simulink model "CLAHEExample"  (R2019b)
settings: Solver=FixedStepDiscrete  StartTime=0.0  StopTime=402*324  FixedStep=1  RelTol=1e-3
PreLoadFcn:
  | % Initialize input image size
  | img = [240 320];
  | 
  | % Number of tiles fixed to 8 x 8
  | numTiles = [8 8];
  | 
  | % Initialize clip limit
  | normClipLimit  = 0.01;
  | 
  | % Number of Bins
  | numBins = 256;
  | 
  | dimI = [240 320] ;
  | 
  | dimTiles = dimI ./ numTiles;
  | 
  | numPixInTile = prod(dimTiles);
  | 
  | minClipLimit = ceil(numPixInTile/numBins);
  | 
  | clipLimit = minClipLimit + round(normClipLimit*(numPixInTile-minClipLimit));
  | 
  | % Initialize value for 1-D lookup table
  | tabVal = uint8(floor(numBins./(1:numBins-1)));
  | 
  | % Initialize wordlength and fractionlength
  | normFact1 = fi(1/(dimTiles(1)*dimTiles(2)/4),0);
  | 
  | normFact2 = fi(1/(prod(dimTiles)/2),0);
  | 
  | normFact3 = fi(1/(prod(dimTiles)),0);
  | 
  | grayxval = (numBins-1)/numPixInTile;
  | fi_grayxval = fi(grayxval,0);
InitFcn:
  | img = imread(get_param('CLAHEExample/inputImage','FileName'));
  | %img = [240 320];
  | numTiles = [8 8];
  | 
  | normClipLimit = str2double(get_param('CLAHEExample/CLAHEHDLAlgorithm','normClipLimit'));
  | 
  | numBins = 256;
  | 
  | dimI = size(img);
  | 
  | dimTiles = dimI ./ numTiles;
  | 
  | numPixInTile = prod(dimTiles);
  | 
  | minClipLimit = ceil(numPixInTile/numBins);
  | 
  | clipLimit = minClipLimit + round(normClipLimit*(numPixInTile-minClipLimit));
  | 
  | tabVal = uint8(floor(numBins./(1:numBins-1)));
  | 
  | normFact1 = fi(1/(dimTiles(1)*dimTiles(2)/4),0);
  | 
  | normFact2 = fi(1/(prod(dimTiles)/2),0);
  | 
  | normFact3 = fi(1/(prod(dimTiles)),0);
  | 
  | grayxval = (numBins-1)/numPixInTile;
  | fi_grayxval = fi(grayxval,0);
libraries: simulink x64, hdlsllib x46, visionhdlutilities x9, visionhdlstatistics x2, visionhdlio x2, visionsources x1
(part 2 of 3)

== system CLAHEExample/CLAHEHDLAlgorithm/tileGeneration/Subsystem ==
  In1 : Inport
  In2 : Inport  Port=2
  In3 : Inport  Port=3
  In4 : Inport  Port=4
  In5 : Inport  Port=5
  In6 : Inport  Port=6
  In7 : Inport  Port=7
  In8 : Inport  Port=8
  In9 : Inport  Port=9
  Multiport Switch{1..5} (5 alike) : MultiPortSwitch  Inputs=8
  Pixel Control Bus Creator : visionhdlutilities/Pixel Control Bus Creator
      settings: SourceProductName=Vision HDL Toolbox  SourceProductBaseCode=VT
  Pixel Control Bus Selector{,1..7} (8 alike) : BusSelector  OutputSignals=hStart,hEnd,vStart,vEnd,valid
  Out1 : Outport  VectorParamsAs1DForOutWhenUnconnected=off
  wires:
  In3/1 -> Pixel Control Bus Selector1/1
  In2/1 -> Pixel Control Bus Selector/1
  In4/1 -> Pixel Control Bus Selector2/1
  Multiport Switch1/1 -> Pixel Control Bus Creator/1
  In5/1 -> Pixel Control Bus Selector3/1
  Pixel Control Bus Creator/1 -> Out1/1
  Pixel Control Bus Selector/1 -> Multiport Switch1/2  "<hStart>"
  Pixel Control Bus Selector1/1 -> Multiport Switch1/3  "<hStart>"
  Pixel Control Bus Selector2/1 -> Multiport Switch1/4  "<hStart>"
  Pixel Control Bus Selector3/1 -> Multiport Switch1/5  "<hStart>"
  Pixel Control Bus Selector4/1 -> Multiport Switch1/6  "<hStart>"
  In6/1 -> Pixel Control Bus Selector4/1
  Pixel Control Bus Selector5/1 -> Multiport Switch1/7  "<hStart>"
  In7/1 -> Pixel Control Bus Selector5/1
  In8/1 -> Pixel Control Bus Selector6/1
  In9/1 -> Pixel Control Bus Selector7/1
  Pixel Control Bus Selector6/1 -> Multiport Switch1/8  "<hStart>"
  Pixel Control Bus Selector7/1 -> Multiport Switch1/9  "<hStart>"
  Pixel Control Bus Selector/2 -> Multiport Switch2/2  "<hEnd>"
  Pixel Control Bus Selector1/2 -> Multiport Switch2/3  "<hEnd>"
  Pixel Control Bus Selector2/2 -> Multiport Switch2/4  "<hEnd>"
  Pixel Control Bus Selector3/2 -> Multiport Switch2/5  "<hEnd>"
  Pixel Control Bus Selector4/2 -> Multiport Switch2/6  "<hEnd>"
  Pixel Control Bus Selector5/2 -> Multiport Switch2/7  "<hEnd>"
  Pixel Control Bus Selector6/2 -> Multiport Switch2/8  "<hEnd>"
  Pixel Control Bus Selector7/2 -> Multiport Switch2/9  "<hEnd>"
  Pixel Control Bus Selector/3 -> Multiport Switch3/2  "<vStart>"
  Pixel Control Bus Selector1/3 -> Multiport Switch3/3  "<vStart>"
  Pixel Control Bus Selector2/3 -> Multiport Switch3/4  "<vStart>"
  Pixel Control Bus Selector3/3 -> Multiport Switch3/5  "<vStart>"
  Pixel Control Bus Selector4/3 -> Multiport Switch3/6  "<vStart>"
  Pixel Control Bus Selector5/3 -> Multiport Switch3/7  "<vStart>"
  Pixel Control Bus Selector6/3 -> Multiport Switch3/8  "<vStart>"
  Pixel Control Bus Selector7/3 -> Multiport Switch3/9  "<vStart>"
  Pixel Control Bus Selector/4 -> Multiport Switch4/2  "<vEnd>"
  Pixel Control Bus Selector1/4 -> Multiport Switch4/3  "<vEnd>"
  Pixel Control Bus Selector2/4 -> Multiport Switch4/4  "<vEnd>"
  Pixel Control Bus Selector3/4 -> Multiport Switch4/5  "<vEnd>"
  Pixel Control Bus Selector4/4 -> Multiport Switch4/6  "<vEnd>"
  Pixel Control Bus Selector5/4 -> Multiport Switch4/7  "<vEnd>"
  Pixel Control Bus Selector6/4 -> Multiport Switch4/8  "<vEnd>"
  Pixel Control Bus Selector7/4 -> Multiport Switch4/9  "<vEnd>"
  Pixel Control Bus Selector/5 -> Multiport Switch5/2  "<valid>"
  Pixel Control Bus Selector1/5 -> Multiport Switch5/3  "<valid>"
  Pixel Control Bus Selector2/5 -> Multiport Switch5/4  "<valid>"
  Pixel Control Bus Selector3/5 -> Multiport Switch5/5  "<valid>"
  Pixel Control Bus Selector4/5 -> Multiport Switch5/6  "<valid>"
  Pixel Control Bus Selector5/5 -> Multiport Switch5/7  "<valid>"
  Pixel Control Bus Selector6/5 -> Multiport Switch5/8  "<valid>"
  Pixel Control Bus Selector7/5 -> Multiport Switch5/9  "<valid>"
  In1/1 -> Multiport Switch2/1, Multiport Switch4/1, Multiport Switch5/1, Multiport Switch3/1, Multiport Switch1/1
  Multiport Switch2/1 -> Pixel Control Bus Creator/2
  Multiport Switch3/1 -> Pixel Control Bus Creator/3
  Multiport Switch4/1 -> Pixel Control Bus Creator/4
  Multiport Switch5/1 -> Pixel Control Bus Creator/5

== system CLAHEExample/CLAHEHDLAlgorithm/tileGeneration/Subsystem1 ==
  Constant : Constant  Value=0  OutDataTypeStr=boolean  SampleTime=-1
  Pixel Control Bus Creator : visionhdlutilities/Pixel Control Bus Creator
      settings: SourceProductName=Vision HDL Toolbox  SourceProductBaseCode=VT
  Out1 : Outport  VectorParamsAs1DForOutWhenUnconnected=off
  wires:
  Constant/1 -> Pixel Control Bus Creator/2, Pixel Control Bus Creator/3, Pixel Control Bus Creator/4, Pixel Control Bus Creator/5, Pixel Control Bus Creator/1
  Pixel Control Bus Creator/1 -> Out1/1

== system CLAHEExample/CLAHEHDLAlgorithm/tileGeneration/VerticalTileExtractor ==
  pixelIn : Inport
  controlIn : Inport  Port=2
  Compare To Constant1 : simulink/Logic and Bit Operations/Compare To Constant  relop===  const=0  OutDataTypeStr=boolean
  Compare To Constant2 : simulink/Logic and Bit Operations/Compare To Constant  relop===  const=dimTiles(1)  OutDataTypeStr=boolean
  Logical Operator1 : Logic  Operator=OR  AllPortsSameDT=off  OutDataTypeStr=boolean
  Logical Operator2 : Logic  Operator=OR  AllPortsSameDT=off  OutDataTypeStr=boolean
  Logical Operator3 : Logic  AllPortsSameDT=off  OutDataTypeStr=boolean
  Logical Operator8 : Logic  AllPortsSameDT=off  OutDataTypeStr=boolean
  Pixel Control Bus Creator : visionhdlutilities/Pixel Control Bus Creator
      settings: SourceProductName=Vision HDL Toolbox  SourceProductBaseCode=VT
  Pixel Control Bus Selector : BusSelector  OutputSignals=hStart,hEnd,vStart,vEnd,valid
  RegionCount : hdlsllib/Sources/HDL Counter  CountType=Count limited  CountInit=0  CountStep=1  CountMax=dimTiles(1)  CountFromType=Initial value  CountFrom=0  CountResetPort=on  CountLoadPort=off  CountEnbPort=on  CountDirPort=off  CountDataType=Unsigned  CountWordLen=ceil(log2(dimTiles(1)))  CountFracLen=0  CountSampTime=1
      settings: SourceProductName=Simulink
  pixelOut : Outport  VectorParamsAs1DForOutWhenUnconnected=off
  controlOut : Outport  Port=2  VectorParamsAs1DForOutWhenUnconnected=off
  wires:
  RegionCount/1 -> Compare To Constant2/1, Compare To Constant1/1
  Pixel Control Bus Selector/4 -> Logical Operator2/1  "<vEnd>"
  Pixel Control Bus Selector/1 -> RegionCount/2, Pixel Control Bus Creator/1, Logical Operator8/2  "<hStart>"
  Pixel Control Bus Selector/2 -> Pixel Control Bus Creator/2, Logical Operator3/2  "<hEnd>"
  pixelIn/1 -> pixelOut/1
  Logical Operator3/1 -> Logical Operator2/2
  Logical Operator1/1 -> Pixel Control Bus Creator/3
  Logical Operator8/1 -> Logical Operator1/1
  Pixel Control Bus Selector/3 -> Logical Operator1/2  "<vStart>"
  Logical Operator2/1 -> Pixel Control Bus Creator/4, RegionCount/1
  Pixel Control Bus Creator/1 -> controlOut/1
  Pixel Control Bus Selector/5 -> Pixel Control Bus Creator/5  "<valid>"
  controlIn/1 -> Pixel Control Bus Selector/1
  Compare To Constant1/1 -> Logical Operator8/1
  Compare To Constant2/1 -> Logical Operator3/1

== system CLAHEExample/CLAHEHDLAlgorithm/tileGeneration/histResetBuffer ==
  pixelIn : Inport
  busIn : Inport  Port=2
  Bus Selector : BusSelector  OutputSignals=valid,vStart
  Delay : Delay  DelayLength=1
  Delay1 : Delay  DelayLength=1
  Delay3 : Delay  DelayLength=numBins
  Delay4 : Delay  DelayLength=numBins
  pixelBusGenerator : Subsystem  mask{hEnd=dimI(2)-1, vEnd=(dimI(1)*dimI(2))-1}
      mask prompts: hEnd "hEnd Count"; vEnd "vEnd Count"
      mask DialogControl DescGroupVar Prompt: Counter Values
  pixelOut : Outport  VectorParamsAs1DForOutWhenUnconnected=off
  busOut : Outport  Port=2  VectorParamsAs1DForOutWhenUnconnected=off
  reset : Outport  Port=3  VectorParamsAs1DForOutWhenUnconnected=off
  wires:
  Delay3/1 -> pixelOut/1
  pixelIn/1 -> Delay/1
  busIn/1 -> Bus Selector/1
  Bus Selector/1 -> Delay1/1  "<valid>"
  Bus Selector/2 -> reset/1, pixelBusGenerator/1(reset)  "<vStart>"
  Delay1/1 -> Delay4/1
  pixelBusGenerator/1(busOut) -> busOut/1
  Delay/1 -> Delay3/1
  Delay4/1 -> pixelBusGenerator/2(validIn)

== system CLAHEExample/CLAHEHDLAlgorithm/bilinearInterpolation/outputStage/pixelBusGenerator ==
  validIn : Inport
  Delay : Delay  DelayLength=1
  Horizontal : hdlsllib/Sources/HDL Counter  CountType=Count limited  CountInit=0  CountStep=1  CountMax=hEnd  CountFromType=Initial value  CountFrom=0  CountResetPort=on  CountLoadPort=off  CountEnbPort=on  CountDirPort=off  CountDataType=Unsigned  CountWordLen=ceil(log2(hEnd))  CountFracLen=0  CountSampTime=1
      settings: SourceProductName=Simulink
  Logical Operator{3..6} (4 alike) : Logic  AllPortsSameDT=off  OutDataTypeStr=boolean
  Pixel Control Bus Creator : visionhdlutilities/Pixel Control Bus Creator
      settings: SourceProductName=Vision HDL Toolbox  SourceProductBaseCode=VT
  Vertical : hdlsllib/Sources/HDL Counter  CountType=Count limited  CountInit=0  CountStep=1  CountMax=vEnd  CountFromType=Initial value  CountFrom=0  CountResetPort=on  CountLoadPort=off  CountEnbPort=on  CountDirPort=off  CountDataType=Unsigned  CountWordLen=ceil(log2(vEnd))  CountFracLen=0  CountSampTime=1
      settings: SourceProductName=Simulink
  hEnd : simulink/Logic and Bit Operations/Compare To Constant  relop===  const=hEnd  OutDataTypeStr=boolean
  hStart : simulink/Logic and Bit Operations/Compare To Constant  relop===  const=0  OutDataTypeStr=boolean
  vEnd : simulink/Logic and Bit Operations/Compare To Constant  relop===  const=vEnd  OutDataTypeStr=boolean
  vStart : simulink/Logic and Bit Operations/Compare To Constant  relop===  const=0  OutDataTypeStr=boolean
  busOut : Outport  VectorParamsAs1DForOutWhenUnconnected=off
  reset : Outport  Port=2  VectorParamsAs1DForOutWhenUnconnected=off
  wires:
  validIn/1 -> Logical Operator4/1, Logical Operator5/1, Logical Operator6/1, Logical Operator3/1, Horizontal/2, Pixel Control Bus Creator/5, Vertical/2
  Horizontal/1 -> hEnd/1, hStart/1
  hEnd/1 -> Logical Operator4/2
  Vertical/1 -> vStart/1, vEnd/1
  vStart/1 -> Logical Operator5/2
  vEnd/1 -> Logical Operator6/2
  Logical Operator5/1 -> Pixel Control Bus Creator/3
  Logical Operator3/1 -> Pixel Control Bus Creator/1
  Logical Operator4/1 -> Pixel Control Bus Creator/2
  hStart/1 -> Logical Operator3/2
  Logical Operator6/1 -> Delay/1, Pixel Control Bus Creator/4
  Pixel Control Bus Creator/1 -> busOut/1
  Delay/1 -> reset/1, Horizontal/1, Vertical/1

== system CLAHEExample/CLAHEHDLAlgorithm/bilinearInterpolation/paramCalc/For Each Subsystem ==
  colCounter : Inport
  Index : Inport  Port=2  Partition=on  PartitionDimension=1  PartitionWidth=1  PartitionOffset=0
  Add : Sum  Inputs=+-
  Add1 : Sum
  Constant : Constant  Value=dimTiles(2)  OutDataTypeStr=fixdt(0,ceil(log2(dimTiles(2))),0)  SampleTime=-1
  Constant1 : Constant  OutDataTypeStr=uint8  SampleTime=-1
  Constant2 : Constant  Value=(dimTiles(2)/2) - 1  OutDataTypeStr=fixdt(0,ceil(log2(dimTiles(2))),0)  SampleTime=-1
  Delay : Delay
  Delay1 : Delay
  For Each : ForEach  DisableCoverage=on
  Product : Product
  Relational Operator : RelationalOperator  Operator===  OutDataTypeStr=boolean  RndMeth=Nearest
  Out1 : Outport  ConcatenationDimension=1  VectorParamsAs1DForOutWhenUnconnected=off
  wires:
  Relational Operator/1 -> Out1/1
  Index/1 -> Add/1
  Add/1 -> Delay1/1
  Constant/1 -> Product/2
  Constant1/1 -> Add/2
  Product/1 -> Delay/1
  Add1/1 -> Relational Operator/2
  Constant2/1 -> Add1/2
  colCounter/1 -> Relational Operator/1
  Delay/1 -> Add1/1
  Delay1/1 -> Product/1

== system CLAHEExample/CLAHEHDLAlgorithm/bilinearInterpolation/paramCalc/For Each Subsystem1 ==
  rowCounter : Inport
  Index : Inport  Port=2  Partition=on  PartitionDimension=1  PartitionWidth=1  PartitionOffset=0
  en : Inport  Port=3
  Add : Sum  Inputs=+-
  Add1 : Sum
  Constant : Constant  Value=dimTiles(1)  OutDataTypeStr=fixdt(0,ceil(log2(dimTiles(1))),0)  SampleTime=-1
  Constant1 : Constant  OutDataTypeStr=uint8  SampleTime=-1
  Constant2 : Constant  Value=(dimTiles(1)/2)-1  OutDataTypeStr=fixdt(0,ceil(log2((dimTiles(1)/2))),0)  SampleTime=-1
  Delay : Delay
  Delay1 : Delay
  For Each : ForEach  DisableCoverage=on
  Logical Operator : Logic  AllPortsSameDT=off  OutDataTypeStr=boolean
  Product : Product
  Relational Operator : RelationalOperator  Operator===  OutDataTypeStr=boolean  RndMeth=Nearest
  Out1 : Outport  ConcatenationDimension=1  VectorParamsAs1DForOutWhenUnconnected=off
  wires:
  Index/1 -> Add/1
  Add/1 -> Delay/1
  Constant/1 -> Product/2
  Constant1/1 -> Add/2
  Product/1 -> Delay1/1
  Add1/1 -> Relational Operator/2
  Constant2/1 -> Add1/2
  rowCounter/1 -> Relational Operator/1
  Relational Operator/1 -> Logical Operator/1
  Logical Operator/1 -> Out1/1
  en/1 -> Logical Operator/2
  Delay/1 -> Product/1
  Delay1/1 -> Add1/1

== system CLAHEExample/CLAHEHDLAlgorithm/bilinearInterpolation/paramCalc/For Each Subsystem2 ==
  rowCounter : Inport
  Index : Inport  Port=2  Partition=on  PartitionDimension=1  PartitionWidth=1  PartitionOffset=0
  en : Inport  Port=3
  Add : Sum  Inputs=+-
  Add1 : Sum
  Constant : Constant  Value=2*dimTiles(1)  OutDataTypeStr=fixdt(0,ceil(log2(2*dimTiles(1))),0)  SampleTime=-1
  Constant1 : Constant  OutDataTypeStr=uint8  SampleTime=-1
  Constant2 : Constant  Value=(dimTiles(1) + dimTiles(1)/2)-1  OutDataTypeStr=fixdt(0,ceil(log2((dimTiles(1) + dimTiles(1)/2))),0)  SampleTime=-1
  Delay : Delay
  Delay1 : Delay
  For Each : ForEach  DisableCoverage=on
  Logical Operator : Logic  AllPortsSameDT=off  OutDataTypeStr=boolean
  Product : Product
  Relational Operator : RelationalOperator  Operator===  OutDataTypeStr=boolean  RndMeth=Nearest
  Out1 : Outport  ConcatenationDimension=1  VectorParamsAs1DForOutWhenUnconnected=off
  wires:
  Index/1 -> Add/1
  Add/1 -> Delay/1
  Constant/1 -> Product/2
  Constant1/1 -> Add/2
  Product/1 -> Delay1/1
  Add1/1 -> Relational Operator/2
  Constant2/1 -> Add1/2
  rowCounter/1 -> Relational Operator/1
  Relational Operator/1 -> Logical Operator/1
  Logical Operator/1 -> Out1/1
  en/1 -> Logical Operator/2
  Delay/1 -> Product/1
  Delay1/1 -> Add1/1

== system CLAHEExample/CLAHEHDLAlgorithm/bilinearInterpolation/paramCalc/For Each Subsystem3 ==
  rowCounter : Inport
  Index : Inport  Port=2  Partition=on  PartitionDimension=1  PartitionWidth=1  PartitionOffset=0
  en : Inport  Port=3
  Add : Sum  Inputs=+-
  Add1 : Sum
  Constant : Constant  Value=2*dimTiles(1)  OutDataTypeStr=fixdt(0,ceil(log2(2*dimTiles(1))),0)  SampleTime=-1
  Constant1 : Constant  OutDataTypeStr=uint8  SampleTime=-1
  Constant2 : Constant  Value=(2*dimTiles(1) + dimTiles(1)/2)-1  OutDataTypeStr=fixdt(0,ceil(log2(2*dimTiles(1) + dimTiles(1))),0)  SampleTime=-1
  Delay : Delay
  Delay1 : Delay
  For Each : ForEach  DisableCoverage=on
  Logical Operator : Logic  AllPortsSameDT=off  OutDataTypeStr=boolean
  Product : Product
  Relational Operator : RelationalOperator  Operator===  OutDataTypeStr=boolean  RndMeth=Nearest
  Out1 : Outport  ConcatenationDimension=1  VectorParamsAs1DForOutWhenUnconnected=off
  wires:
  Index/1 -> Add/1
  Add/1 -> Delay/1
  Constant/1 -> Product/2
  Constant1/1 -> Add/2
  Product/1 -> Delay1/1
  Add1/1 -> Relational Operator/2
  Constant2/1 -> Add1/2
  rowCounter/1 -> Relational Operator/1
  Relational Operator/1 -> Logical Operator/1
  Logical Operator/1 -> Out1/1
  en/1 -> Logical Operator/2
  Delay/1 -> Product/1
  Delay1/1 -> Add1/1

== system CLAHEExample/CLAHEHDLAlgorithm/bilinearInterpolation/paramCalc/pixelBusGenerator ==
  validIn : Inport
  Horizontal : hdlsllib/Sources/HDL Counter  CountType=Count limited  CountInit=0  CountStep=1  CountMax=hEnd  CountFromType=Initial value  CountFrom=0  CountResetPort=off  CountLoadPort=off  CountEnbPort=on  CountDirPort=off  CountDataType=Unsigned  CountWordLen=ceil(log2(hEnd))  CountFracLen=0  CountSampTime=1
      settings: SourceProductName=Simulink
  Logical Operator{3..6} (4 alike) : Logic  AllPortsSameDT=off  OutDataTypeStr=boolean
  Pixel Control Bus Creator : visionhdlutilities/Pixel Control Bus Creator
      settings: SourceProductName=Vision HDL Toolbox  SourceProductBaseCode=VT
  Vertical : hdlsllib/Sources/HDL Counter  CountType=Count limited  CountInit=0  CountStep=1  CountMax=vEnd  CountFromType=Initial value  CountFrom=0  CountResetPort=off  CountLoadPort=off  CountEnbPort=on  CountDirPort=off  CountDataType=Unsigned  CountWordLen=ceil(log2(vEnd))  CountFracLen=0  CountSampTime=1
      settings: SourceProductName=Simulink
  hEnd : simulink/Logic and Bit Operations/Compare To Constant  relop===  const=hEnd  OutDataTypeStr=boolean
  hStart : simulink/Logic and Bit Operations/Compare To Constant  relop===  const=0  OutDataTypeStr=boolean
  vEnd : simulink/Logic and Bit Operations/Compare To Constant  relop===  const=vEnd  OutDataTypeStr=boolean
  vStart : simulink/Logic and Bit Operations/Compare To Constant  relop===  const=0  OutDataTypeStr=boolean
  busOut : Outport  VectorParamsAs1DForOutWhenUnconnected=off
  frameDone : Outport  Port=2  VectorParamsAs1DForOutWhenUnconnected=off
  wires:
  validIn/1 -> Pixel Control Bus Creator/5, Vertical/1, Logical Operator4/1, Logical Operator5/1, Logical Operator6/1, Logical Operator3/1, Horizontal/1
  Horizontal/1 -> hEnd/1, hStart/1
  hEnd/1 -> Logical Operator4/2
  Vertical/1 -> vStart/1, vEnd/1
  vStart/1 -> Logical Operator5/2
  vEnd/1 -> Logical Operator6/2
  Logical Operator5/1 -> Pixel Control Bus Creator/3
  Logical Operator3/1 -> Pixel Control Bus Creator/1
  Logical Operator4/1 -> Pixel Control Bus Creator/2
  hStart/1 -> Logical Operator3/2
  Logical Operator6/1 -> frameDone/1, Pixel Control Bus Creator/4
  Pixel Control Bus Creator/1 -> busOut/1

== system CLAHEExample/CLAHEHDLAlgorithm/histoEqPipeline/histPipe1/cdf ==
  histoIn : Inport
  valid : Inport  Port=2
  active : Inport  Port=3
  Add : Sum  OutDataTypeStr=fixdt(0,ceil(log2(numPixInTile)),0)
  Bus Creator : BusCreator  Inputs=5
  Compare To Constant : simulink/Logic and Bit Operations/Compare To Constant  relop=<  const=256  OutDataTypeStr=boolean
  Compare To Constant1 : simulink/Logic and Bit Operations/Compare To Constant  relop===  const=255  OutDataTypeStr=boolean
  Constant : Constant  Value=0  OutDataTypeStr=fixdt(0,9,0)  SampleTime=-1
  Constant1 : Constant  Value=0  OutDataTypeStr=boolean  SampleTime=-1
  Constant2 : Constant  Value=0  OutDataTypeStr=fixdt(0,ceil(log2(numPixInTile)),0)  SampleTime=-1
  Data Type Conversion : DataTypeConversion  OutDataTypeStr=uint8
  Delay{,1..3} (4 alike) : Delay  DelayLength=1
  HDL Counter : hdlsllib/Sources/HDL Counter  CountType=Free running  CountInit=0  CountStep=1  CountMax=255  CountFromType=Initial value  CountFrom=0  CountResetPort=on  CountLoadPort=off  CountEnbPort=on  CountDirPort=off  CountDataType=Unsigned  CountWordLen=9  CountFracLen=0  CountSampTime=1
      settings: SourceProductName=Simulink
  Switch : Switch  Criteria=u2 ~= 0
  Switch1 : Switch  Criteria=u2 ~= 0
  Switch2 : Switch  Criteria=u2 ~= 0
  ramBus : Outport  VectorParamsAs1DForOutWhenUnconnected=off
  done : Outport  Port=2  VectorParamsAs1DForOutWhenUnconnected=off
  wires:
  Bus Creator/1 -> ramBus/1
  Compare To Constant1/1 -> HDL Counter/1, done/1
  histoIn/1 -> Add/1
  Add/1 -> Delay/1, Bus Creator/1  "histVal"
  Compare To Constant/1 -> Switch1/2, Switch/2
  HDL Counter/1 -> Switch/1, Compare To Constant/1
  Constant/1 -> Switch/3
  Switch/1 -> Data Type Conversion/1
  Data Type Conversion/1 -> Delay2/1, Bus Creator/4  "rd_addr"
  active/1 -> Switch1/1, HDL Counter/2  "rd_valid"
  Delay2/1 -> Compare To Constant1/1, Bus Creator/2  "wr_addr"
  Delay3/1 -> Bus Creator/3  "wr_en"
  Constant1/1 -> Switch1/3
  Switch1/1 -> Delay3/1, Bus Creator/5  "rd_valid"
  valid/1 -> Delay1/1
  Switch2/1 -> Add/2
  Delay/1 -> Switch2/1
  Constant2/1 -> Switch2/3
  Delay1/1 -> Switch2/2

== system CLAHEExample/CLAHEHDLAlgorithm/histoEqPipeline/histPipe1/cdfRefresh ==
  frameDone : Inport
  Add : Sum  Inputs=+-  OutDataTypeStr=uint8
  Compare To Constant3 : simulink/Logic and Bit Operations/Compare To Constant  relop=>  const=0  OutDataTypeStr=boolean
  Compare To Constant4 : simulink/Logic and Bit Operations/Compare To Constant  relop=<=  const=numBins  OutDataTypeStr=boolean
  Compare To Constant5 : simulink/Logic and Bit Operations/Compare To Constant  relop=>  const=0  OutDataTypeStr=boolean
  Compare To Constant7 : simulink/Logic and Bit Operations/Compare To Constant  relop===  const=numBins+5  OutDataTypeStr=boolean
  Constant : Constant  Value=0  OutDataTypeStr=uint8  SampleTime=-1
  Constant3 : Constant  OutDataTypeStr=uint8  SampleTime=-1
  Delay : Delay  DelayLength=1
  HDL Counter2 : hdlsllib/Sources/HDL Counter  CountType=Count limited  CountInit=0  CountStep=1  CountMax=(numBins*2)-1  CountFromType=Initial value  CountFrom=0  CountResetPort=on  CountLoadPort=off  CountEnbPort=on  CountDirPort=off  CountDataType=Unsigned  CountWordLen=ceil(log2(numBins*2))  CountFracLen=0  CountSampTime=1
      settings: SourceProductName=Simulink
  HDL Counter4 : hdlsllib/Sources/HDL Counter  CountType=Count limited  CountInit=0  CountStep=1  CountMax=(numBins*2)-1  CountFromType=Initial value  CountFrom=0  CountResetPort=on  CountLoadPort=off  CountEnbPort=on  CountDirPort=off  CountDataType=Unsigned  CountWordLen=ceil(log2(numBins*2))  CountFracLen=0  CountSampTime=1
      settings: SourceProductName=Simulink
  HDL Counter6 : hdlsllib/Sources/HDL Counter  CountType=Count limited  CountInit=1  CountStep=1  CountMax=2  CountFromType=Initial value  CountFrom=1  CountResetPort=off  CountLoadPort=off  CountEnbPort=on  CountDirPort=off  CountDataType=Unsigned  CountWordLen=3  CountFracLen=0  CountSampTime=1
      settings: SourceProductName=Simulink
  Logical Operator3 : Logic  AllPortsSameDT=off  OutDataTypeStr=boolean
  Logical Operator4 : Logic  Operator=OR  AllPortsSameDT=off  OutDataTypeStr=boolean
  histVal : Outport
  wr_addr : Outport  Port=2
  wr_en : Outport  Port=3
  rd_addr : Outport  Port=4
  select : Outport  Port=5
  wires:
  Compare To Constant4/1 -> Logical Operator3/2
  frameDone/1 -> HDL Counter4/2, Logical Operator4/1
  Constant3/1 -> Add/2
  Compare To Constant7/1 -> HDL Counter2/1, HDL Counter4/1, Logical Operator4/2
  HDL Counter2/1 -> Compare To Constant7/1, Add/1, Compare To Constant3/1, Compare To Constant4/1
  Logical Operator4/1 -> HDL Counter6/1
  HDL Counter6/1 -> select/1
  Constant/1 -> histVal/1, Delay/1
  HDL Counter4/1 -> Compare To Constant5/1
  Compare To Constant5/1 -> HDL Counter2/2
  Compare To Constant3/1 -> Logical Operator3/1
  Delay/1 -> rd_addr/1
  Logical Operator3/1 -> wr_en/1  "wr_en"
  Add/1 -> wr_addr/1  "wr_addr"

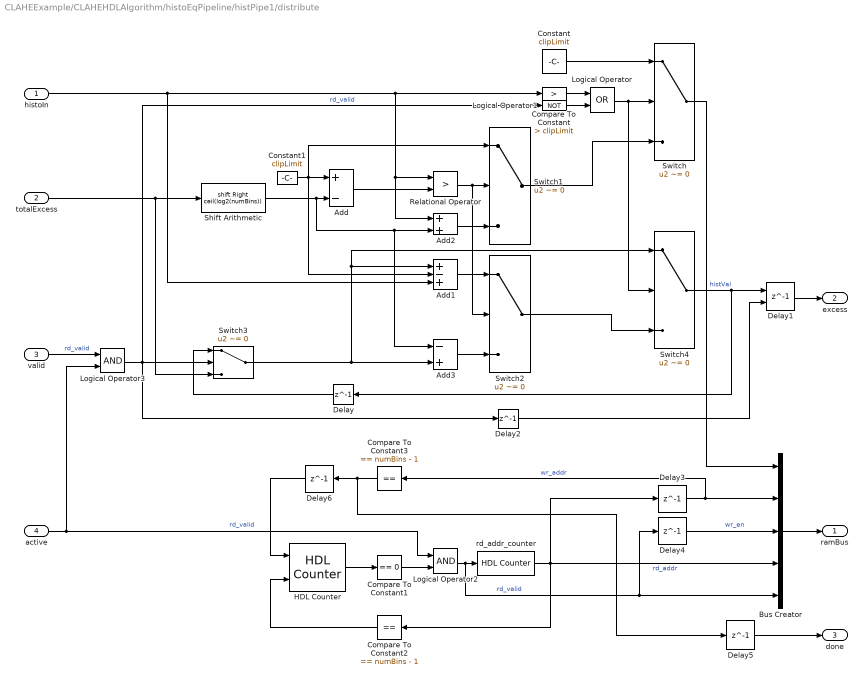
== system CLAHEExample/CLAHEHDLAlgorithm/histoEqPipeline/histPipe1/distribute ==
  histoIn : Inport
  totalExcess : Inport  Port=2
  valid : Inport  Port=3
  active : Inport  Port=4
  Add : Sum  Inputs=+-  OutDataTypeStr=fixdt(0,ceil(log2(numPixInTile)),0)
  Add1 : Sum  Inputs=+-+
  Add2 : Sum  OutDataTypeStr=fixdt(0,ceil(log2(numPixInTile)),0)
  Add3 : Sum  Inputs=-+
  Bus Creator : BusCreator  Inputs=5
  Compare To Constant : simulink/Logic and Bit Operations/Compare To Constant  relop=>  const=clipLimit  OutDataTypeStr=boolean
  Compare To Constant1 : simulink/Logic and Bit Operations/Compare To Constant  relop===  const=0  OutDataTypeStr=boolean
  Compare To Constant2 : simulink/Logic and Bit Operations/Compare To Constant  relop===  const=numBins - 1  OutDataTypeStr=boolean
  Compare To Constant3 : simulink/Logic and Bit Operations/Compare To Constant  relop===  const=numBins - 1  OutDataTypeStr=boolean
  Constant : Constant  Value=clipLimit  OutDataTypeStr=fixdt(0,ceil(log2(numPixInTile)),0)  SampleTime=-1
  Constant1 : Constant  Value=clipLimit  OutDataTypeStr=fixdt(0,ceil(log2(numPixInTile)),0)  SampleTime=-1
  Delay{,2..6} (6 alike) : Delay  DelayLength=1
  Delay1 : Delay  DelayLength=1  InitialCondition=255  ShowEnablePort=on
      settings: InputPortMap=u0,e6
  HDL Counter : hdlsllib/Sources/HDL Counter  CountType=Count limited  CountInit=0  CountStep=1  CountMax=3  CountFromType=Initial value  CountFrom=0  CountResetPort=on  CountLoadPort=off  CountEnbPort=on  CountDirPort=off  CountDataType=Unsigned  CountWordLen=2  CountFracLen=0  CountSampTime=1
      settings: SourceProductName=Simulink
  Logical Operator : Logic  Operator=OR  AllPortsSameDT=off  OutDataTypeStr=boolean
  Logical Operator1 : Logic  Operator=NOT  AllPortsSameDT=off  OutDataTypeStr=boolean
  Logical Operator2 : Logic  AllPortsSameDT=off  OutDataTypeStr=boolean
  Logical Operator3 : Logic  AllPortsSameDT=off  OutDataTypeStr=boolean
  Relational Operator : RelationalOperator  Operator=>  OutDataTypeStr=boolean  RndMeth=Nearest
  Shift Arithmetic : ArithShift  BitShiftNumber=ceil(log2(numBins))  BitShiftDirection=Right
  Switch{,1..4} (5 alike) : Switch  Criteria=u2 ~= 0
  rd_addr_counter : hdlsllib/Sources/HDL Counter  CountType=Free running  CountInit=0  CountStep=1  CountMax=255  CountFromType=Initial value  CountFrom=0  CountResetPort=off  CountLoadPort=off  CountEnbPort=on  CountDirPort=off  CountDataType=Unsigned  CountWordLen=ceil(log2(numBins))  CountFracLen=0  CountSampTime=1
      settings: SourceProductName=Simulink
  ramBus : Outport  VectorParamsAs1DForOutWhenUnconnected=off
  excess : Outport  Port=2  VectorParamsAs1DForOutWhenUnconnected=off
  done : Outport  Port=3  VectorParamsAs1DForOutWhenUnconnected=off
  wires:
  Constant/1 -> Switch/1
  totalExcess/1 -> Switch3/3, Shift Arithmetic/1
  Shift Arithmetic/1 -> Add3/1, Add2/2, Add/2
  Constant1/1 -> Switch1/1, Add1/2, Add/1
  Relational Operator/1 -> Switch2/2, Switch1/2
  histoIn/1 -> Add1/3, Add2/1, Relational Operator/1, Compare To Constant/1
  Add/1 -> Relational Operator/2
  Add2/1 -> Switch1/3
  Add1/1 -> Switch2/1
  Add3/1 -> Switch2/3
  Switch1/1 -> Switch/3
  Switch3/1 -> Switch4/1, Add1/1, Add3/2
  Delay/1 -> Switch3/1
  Switch4/1 -> Delay1/1, Delay/1
  Switch2/1 -> Switch4/3
  Delay1/1 -> excess/1
  Delay2/1 -> Delay1/2
  Compare To Constant/1 -> Logical Operator/1
  Logical Operator/1 -> Switch4/2, Switch/2
  Logical Operator1/1 -> Logical Operator/2
  Delay4/1 -> Bus Creator/3  "wr_en"
  Bus Creator/1 -> ramBus/1
  Delay3/1 -> Compare To Constant3/1, Bus Creator/2  "wr_addr"
  Logical Operator3/1 -> Delay2/1, Logical Operator1/1, Switch3/2  "rd_valid"
  Switch/1 -> Bus Creator/1  "histVal"
  rd_addr_counter/1 -> Delay3/1, Bus Creator/4, Compare To Constant2/1  "rd_addr"
  HDL Counter/1 -> Compare To Constant1/1
  Logical Operator2/1 -> Delay4/1, Bus Creator/5, rd_addr_counter/1  "rd_valid"
  Compare To Constant1/1 -> Logical Operator2/2
  Compare To Constant2/1 -> HDL Counter/2
  Compare To Constant3/1 -> Delay5/1, Delay6/1
  Delay5/1 -> done/1
  Delay6/1 -> HDL Counter/1
  active/1 -> Logical Operator3/2, Logical Operator2/1  "rd_valid"
  valid/1 -> Logical Operator3/1  "rd_valid"

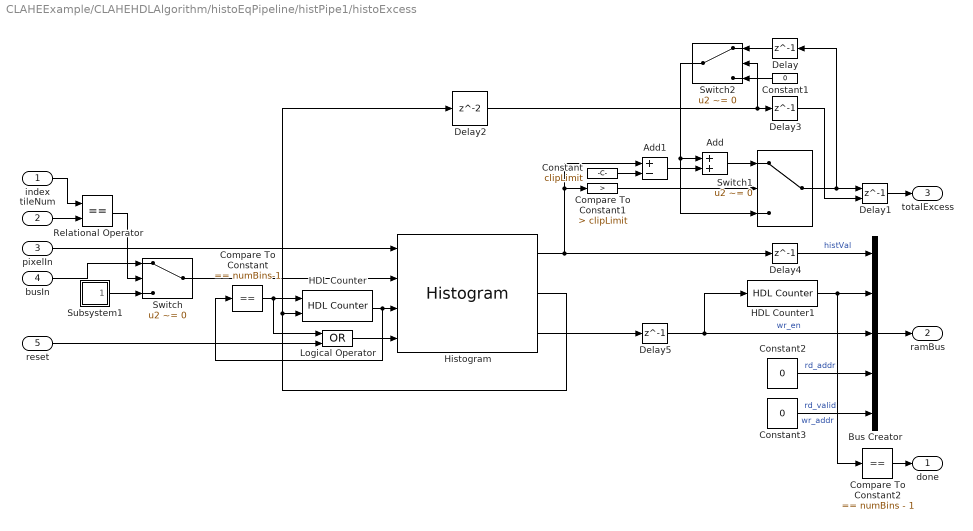
== system CLAHEExample/CLAHEHDLAlgorithm/histoEqPipeline/histPipe1/histoExcess ==
  index : Inport
  tileNum : Inport  Port=2
  pixelIn : Inport  Port=3
  busIn : Inport  Port=4
  reset : Inport  Port=5
  Add : Sum  OutDataTypeStr=fixdt(0,ceil(log2(numPixInTile)),0)
  Add1 : Sum  Inputs=+-
  Bus Creator : BusCreator  Inputs=5
  Compare To Constant : simulink/Logic and Bit Operations/Compare To Constant  relop===  const=numBins-1  OutDataTypeStr=boolean
  Compare To Constant1 : simulink/Logic and Bit Operations/Compare To Constant  relop=>  const=clipLimit  OutDataTypeStr=boolean
  Compare To Constant2 : simulink/Logic and Bit Operations/Compare To Constant  relop===  const=numBins - 1  OutDataTypeStr=boolean
  Constant : Constant  Value=clipLimit  OutDataTypeStr=fixdt(0,ceil(log2(numPixInTile)),0)  SampleTime=-1
  Constant1 : Constant  Value=0  OutDataTypeStr=fixdt(0,ceil(log2(numPixInTile)),0)  SampleTime=-1
  Constant2 : Constant  Value=0  OutDataTypeStr=uint8  SampleTime=-1
  Constant3 : Constant  Value=0  OutDataTypeStr=boolean  SampleTime=-1
  Delay{,3..5} (4 alike) : Delay  DelayLength=1
  Delay1 : Delay  DelayLength=1  ShowEnablePort=on
      settings: InputPortMap=u0,e6
  Delay2 : Delay
  HDL Counter : hdlsllib/Sources/HDL Counter  CountType=Count limited  CountInit=0  CountStep=1  CountMax=numBins-1  CountFromType=Initial value  CountFrom=0  CountResetPort=on  CountLoadPort=off  CountEnbPort=on  CountDirPort=off  CountDataType=Unsigned  CountWordLen=ceil(log2(numBins))  CountFracLen=0  CountSampTime=1
      settings: SourceProductName=Simulink
  HDL Counter1 : hdlsllib/Sources/HDL Counter  CountType=Count limited  CountInit=0  CountStep=1  CountMax=numBins - 1  CountFromType=Initial value  CountFrom=0  CountResetPort=off  CountLoadPort=off  CountEnbPort=on  CountDirPort=off  CountDataType=Unsigned  CountWordLen=ceil(log2(numBins))  CountFracLen=0  CountSampTime=1
      settings: SourceProductName=Simulink
  Histogram : visionhdlstatistics/Histogram  NumBins=256  OutputDataType=Unsigned fixed point  OutputWL=ceil(log2(numPixInTile))  SimulateUsing=Code generation
      settings: SourceProductName=Vision HDL Toolbox  SourceProductBaseCode=VT
  Logical Operator : Logic  Operator=OR  AllPortsSameDT=off  OutDataTypeStr=boolean
  Relational Operator : RelationalOperator  Operator===  OutDataTypeStr=boolean  RndMeth=Nearest
  Subsystem1 : Subsystem
  Switch : Switch  Criteria=u2 ~= 0
  Switch1 : Switch  Criteria=u2 ~= 0
  Switch2 : Switch  Criteria=u2 ~= 0
  done : Outport  VectorParamsAs1DForOutWhenUnconnected=off
  ramBus : Outport  Port=2  VectorParamsAs1DForOutWhenUnconnected=off
  totalExcess : Outport  Port=3  VectorParamsAs1DForOutWhenUnconnected=off
  wires:
  HDL Counter/1 -> Compare To Constant/1, Histogram/3
  Histogram/2 -> Delay2/1, HDL Counter/2
  Delay2/1 -> Switch2/2, Delay3/1
  Logical Operator/1 -> Histogram/4
  Constant/1 -> Add1/2
  Switch1/1 -> Delay1/1, Delay/1
  reset/1 -> Logical Operator/2
  Add/1 -> Switch1/1
  Compare To Constant1/1 -> Switch1/2
  Add1/1 -> Add/2
  Switch2/1 -> Switch1/3, Add/1
  Delay/1 -> Switch2/1
  Histogram/1 -> Delay4/1, Add1/1, Compare To Constant1/1
  Compare To Constant/1 -> Logical Operator/1, HDL Counter/1
  Constant1/1 -> Switch2/3
  pixelIn/1 -> Histogram/1
  Histogram/3 -> Delay5/1
  Delay5/1 -> Bus Creator/3, HDL Counter1/1  "wr_en"
  Delay4/1 -> Bus Creator/1  "histVal"
  HDL Counter1/1 -> Bus Creator/2, Compare To Constant2/1  "wr_addr"
  Constant2/1 -> Bus Creator/4  "rd_addr"
  Constant3/1 -> Bus Creator/5  "rd_valid"
  Bus Creator/1 -> ramBus/1
  Delay1/1 -> totalExcess/1
  Compare To Constant2/1 -> done/1
  busIn/1 -> Switch/1
  Subsystem1/1(Out1) -> Switch/3
  tileNum/1 -> Relational Operator/2
  index/1 -> Relational Operator/1
  Switch/1 -> Histogram/2
  Relational Operator/1 -> Switch/2
  Delay3/1 -> Delay1/2

== system CLAHEExample/CLAHEHDLAlgorithm/histoEqPipeline/histPipe1/redistribute ==
  histoIn : Inport
  totalExcess : Inport  Port=2
  active : Inport  Port=3
  valid : Inport  Port=4
  1-D Lookup Table1 : Lookup_n-D  NumberOfTableDimensions=1  LookupTableObject=''  BreakpointsForDimension1=[1:255]  BreakpointsForDimension1FirstPoint=10  BreakpointsForDimension2FirstPoint=10  BreakpointsForDimension1Spacing=12  BreakpointsForDimension2Spacing=12  IndexSearchMethod=Evenly spaced points  Table=tabVal  InterpMethod=Flat  DiagnosticForOutOfRangeInput=Error  RemoveProtectionInput=on  InternalRulePriority=Speed  OutDataTypeStr=uint8  RndMeth=Simplest  SaturateOnIntegerOverflow=on  InputSameDT=on
  Add : Sum  OutDataTypeStr=fixdt(0,ceil(log2(numPixInTile)),0)
  Add1 : Sum  Inputs=-+
  Bus Creator : BusCreator  Inputs=5
  Compare To Constant1 : simulink/Logic and Bit Operations/Compare To Constant  relop=<  const=clipLimit  OutDataTypeStr=boolean
  Data Type Conversion : DataTypeConversion  OutDataTypeStr=uint8
  Delay{,1,3,5} (4 alike) : Delay  DelayLength=1
  Logical Operator3 : Logic  AllPortsSameDT=off  OutDataTypeStr=boolean
  Logical Operator4 : Logic  AllPortsSameDT=off  OutDataTypeStr=boolean
  MATLAB Function1 : MATLAB Function  TreatAsAtomicUnit=on
  Switch : Switch  Criteria=u2 ~= 0
  Switch1 : Switch  Criteria=u2 ~= 0
  excessFeedback : Switch  Criteria=u2 ~= 0
  ramBus : Outport  VectorParamsAs1DForOutWhenUnconnected=off
  done : Outport  Port=2  VectorParamsAs1DForOutWhenUnconnected=off
  wires:
  Add/1 -> Switch/1
  Add1/1 -> Switch1/1
  totalExcess/1 -> excessFeedback/3
  excessFeedback/1 -> MATLAB Function1/2(excessIn), Switch1/3, Add1/2
  Delay/1 -> excessFeedback/1
  Switch1/1 -> Delay/1
  histoIn/1 -> Add/1, Switch/3, Compare To Constant1/1
  Bus Creator/1 -> ramBus/1
  Delay3/1 -> Bus Creator/3  "wr_en"
  Delay5/1 -> Bus Creator/2  "wr_addr"
  MATLAB Function1/4(done) -> done/1
  MATLAB Function1/3(rdValid) -> Bus Creator/5, Delay3/1  "rd_valid"
  MATLAB Function1/2(rdAddr) -> Bus Creator/4, Delay5/1  "rd_addr"
  Compare To Constant1/1 -> Logical Operator3/1
  Logical Operator3/1 -> Switch/2, Switch1/2
  valid/1 -> Logical Operator4/1
  Logical Operator4/1 -> Logical Operator3/2
  active/1 -> MATLAB Function1/1(active), Logical Operator4/2, excessFeedback/2
  MATLAB Function1/1(binIncr) -> Add1/1, Add/2
  MATLAB Function1/5(excessOut) -> Data Type Conversion/1
  1-D Lookup Table1/1 -> Delay1/1
  Delay1/1 -> MATLAB Function1/3(stepIn)
  Data Type Conversion/1 -> 1-D Lookup Table1/1
  Switch/1 -> Bus Creator/1  "histVal"

== system CLAHEExample/CLAHEHDLAlgorithm/histoEqPipeline/histPipe2/cdf ==
  histoIn : Inport
  valid : Inport  Port=2
  active : Inport  Port=3
  Add : Sum  OutDataTypeStr=fixdt(0,ceil(log2(numPixInTile)),0)
  Bus Creator : BusCreator  Inputs=5
  Compare To Constant : simulink/Logic and Bit Operations/Compare To Constant  relop=<  const=256  OutDataTypeStr=boolean
  Compare To Constant1 : simulink/Logic and Bit Operations/Compare To Constant  relop===  const=255  OutDataTypeStr=boolean
  Constant : Constant  Value=0  OutDataTypeStr=fixdt(0,9,0)  SampleTime=-1
  Constant1 : Constant  Value=0  OutDataTypeStr=boolean  SampleTime=-1
  Constant2 : Constant  Value=0  OutDataTypeStr=fixdt(0,ceil(log2(numPixInTile)),0)  SampleTime=-1
  Data Type Conversion : DataTypeConversion  OutDataTypeStr=uint8
  Delay{,1..3} (4 alike) : Delay  DelayLength=1
  HDL Counter : hdlsllib/Sources/HDL Counter  CountType=Free running  CountInit=0  CountStep=1  CountMax=255  CountFromType=Initial value  CountFrom=0  CountResetPort=on  CountLoadPort=off  CountEnbPort=on  CountDirPort=off  CountDataType=Unsigned  CountWordLen=9  CountFracLen=0  CountSampTime=1
      settings: SourceProductName=Simulink
  Switch : Switch  Criteria=u2 ~= 0
  Switch1 : Switch  Criteria=u2 ~= 0
  Switch2 : Switch  Criteria=u2 ~= 0
  ramBus : Outport  VectorParamsAs1DForOutWhenUnconnected=off
  done : Outport  Port=2  VectorParamsAs1DForOutWhenUnconnected=off
  wires:
  Bus Creator/1 -> ramBus/1
  Compare To Constant1/1 -> HDL Counter/1, done/1
  histoIn/1 -> Add/1
  Add/1 -> Delay/1, Bus Creator/1  "histVal"
  Compare To Constant/1 -> Switch1/2, Switch/2
  HDL Counter/1 -> Switch/1, Compare To Constant/1
  Constant/1 -> Switch/3
  Switch/1 -> Data Type Conversion/1
  Data Type Conversion/1 -> Bus Creator/4, Delay2/1  "rd_addr"
  active/1 -> Switch1/1, HDL Counter/2  "rd_valid"
  Delay2/1 -> Compare To Constant1/1, Bus Creator/2  "wr_addr"
  Delay3/1 -> Bus Creator/3  "wr_en"
  Constant1/1 -> Switch1/3
  Switch1/1 -> Delay3/1, Bus Creator/5  "rd_valid"
  valid/1 -> Delay1/1
  Switch2/1 -> Add/2
  Delay/1 -> Switch2/1
  Constant2/1 -> Switch2/3
  Delay1/1 -> Switch2/2

== system CLAHEExample/CLAHEHDLAlgorithm/histoEqPipeline/histPipe2/cdfRefresh ==
  frameDone : Inport
  Add : Sum  Inputs=+-  OutDataTypeStr=uint8
  Compare To Constant3 : simulink/Logic and Bit Operations/Compare To Constant  relop=>  const=0  OutDataTypeStr=boolean
  Compare To Constant4 : simulink/Logic and Bit Operations/Compare To Constant  relop=<=  const=numBins  OutDataTypeStr=boolean
  Compare To Constant5 : simulink/Logic and Bit Operations/Compare To Constant  relop=>  const=0  OutDataTypeStr=boolean
  Compare To Constant7 : simulink/Logic and Bit Operations/Compare To Constant  relop===  const=numBins+5  OutDataTypeStr=boolean
  Constant : Constant  Value=0  OutDataTypeStr=uint8  SampleTime=-1
  Constant3 : Constant  OutDataTypeStr=uint8  SampleTime=-1
  Delay : Delay  DelayLength=1
  HDL Counter2 : hdlsllib/Sources/HDL Counter  CountType=Count limited  CountInit=0  CountStep=1  CountMax=(numBins*2)-1  CountFromType=Initial value  CountFrom=0  CountResetPort=on  CountLoadPort=off  CountEnbPort=on  CountDirPort=off  CountDataType=Unsigned  CountWordLen=ceil(log2(numBins*2))  CountFracLen=0  CountSampTime=1
      settings: SourceProductName=Simulink
  HDL Counter4 : hdlsllib/Sources/HDL Counter  CountType=Count limited  CountInit=0  CountStep=1  CountMax=(numBins*2)-1  CountFromType=Initial value  CountFrom=0  CountResetPort=on  CountLoadPort=off  CountEnbPort=on  CountDirPort=off  CountDataType=Unsigned  CountWordLen=ceil(log2(numBins*2))  CountFracLen=0  CountSampTime=1
      settings: SourceProductName=Simulink
  HDL Counter6 : hdlsllib/Sources/HDL Counter  CountType=Count limited  CountInit=1  CountStep=1  CountMax=2  CountFromType=Initial value  CountFrom=1  CountResetPort=off  CountLoadPort=off  CountEnbPort=on  CountDirPort=off  CountDataType=Unsigned  CountWordLen=3  CountFracLen=0  CountSampTime=1
      settings: SourceProductName=Simulink
  Logical Operator3 : Logic  AllPortsSameDT=off  OutDataTypeStr=boolean
  Logical Operator4 : Logic  Operator=OR  AllPortsSameDT=off  OutDataTypeStr=boolean
  histVal : Outport
  wr_addr : Outport  Port=2
  wr_en : Outport  Port=3
  rd_addr : Outport  Port=4
  select : Outport  Port=5
  wires:
  Compare To Constant4/1 -> Logical Operator3/2
  frameDone/1 -> HDL Counter4/2, Logical Operator4/1
  Constant3/1 -> Add/2
  Compare To Constant7/1 -> HDL Counter2/1, HDL Counter4/1, Logical Operator4/2
  HDL Counter2/1 -> Compare To Constant7/1, Add/1, Compare To Constant3/1, Compare To Constant4/1
  Logical Operator4/1 -> HDL Counter6/1
  HDL Counter6/1 -> select/1
  Constant/1 -> histVal/1, Delay/1
  HDL Counter4/1 -> Compare To Constant5/1
  Compare To Constant5/1 -> HDL Counter2/2
  Compare To Constant3/1 -> Logical Operator3/1
  Delay/1 -> rd_addr/1
  Logical Operator3/1 -> wr_en/1  "wr_en"
  Add/1 -> wr_addr/1  "wr_addr"

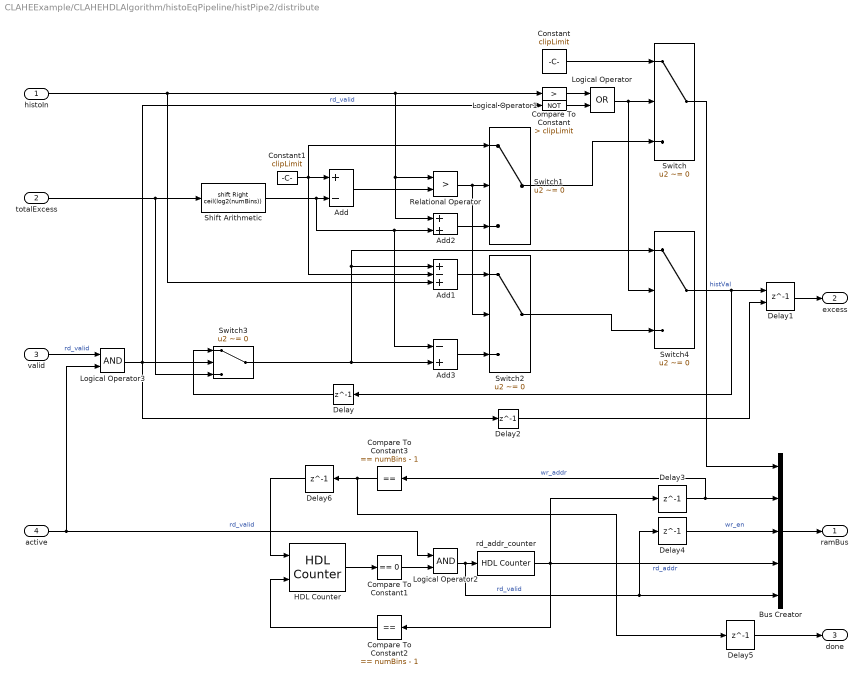
== system CLAHEExample/CLAHEHDLAlgorithm/histoEqPipeline/histPipe2/distribute ==
  histoIn : Inport
  totalExcess : Inport  Port=2
  valid : Inport  Port=3
  active : Inport  Port=4
  Add : Sum  Inputs=+-  OutDataTypeStr=fixdt(0,ceil(log2(numPixInTile)),0)
  Add1 : Sum  Inputs=+-+
  Add2 : Sum  OutDataTypeStr=fixdt(0,ceil(log2(numPixInTile)),0)
  Add3 : Sum  Inputs=-+
  Bus Creator : BusCreator  Inputs=5
  Compare To Constant : simulink/Logic and Bit Operations/Compare To Constant  relop=>  const=clipLimit  OutDataTypeStr=boolean
  Compare To Constant1 : simulink/Logic and Bit Operations/Compare To Constant  relop===  const=0  OutDataTypeStr=boolean
  Compare To Constant2 : simulink/Logic and Bit Operations/Compare To Constant  relop===  const=numBins - 1  OutDataTypeStr=boolean
  Compare To Constant3 : simulink/Logic and Bit Operations/Compare To Constant  relop===  const=numBins - 1  OutDataTypeStr=boolean
  Constant : Constant  Value=clipLimit  OutDataTypeStr=fixdt(0,ceil(log2(numPixInTile)),0)  SampleTime=-1
  Constant1 : Constant  Value=clipLimit  OutDataTypeStr=fixdt(0,ceil(log2(numPixInTile)),0)  SampleTime=-1
  Delay{,2..6} (6 alike) : Delay  DelayLength=1
  Delay1 : Delay  DelayLength=1  InitialCondition=255  ShowEnablePort=on
      settings: InputPortMap=u0,e6
  HDL Counter : hdlsllib/Sources/HDL Counter  CountType=Count limited  CountInit=0  CountStep=1  CountMax=3  CountFromType=Initial value  CountFrom=0  CountResetPort=on  CountLoadPort=off  CountEnbPort=on  CountDirPort=off  CountDataType=Unsigned  CountWordLen=2  CountFracLen=0  CountSampTime=1
      settings: SourceProductName=Simulink
  Logical Operator : Logic  Operator=OR  AllPortsSameDT=off  OutDataTypeStr=boolean
  Logical Operator1 : Logic  Operator=NOT  AllPortsSameDT=off  OutDataTypeStr=boolean
  Logical Operator2 : Logic  AllPortsSameDT=off  OutDataTypeStr=boolean
  Logical Operator3 : Logic  AllPortsSameDT=off  OutDataTypeStr=boolean
  Relational Operator : RelationalOperator  Operator=>  OutDataTypeStr=boolean  RndMeth=Nearest
  Shift Arithmetic : ArithShift  BitShiftNumber=ceil(log2(numBins))  BitShiftDirection=Right
  Switch{,1..4} (5 alike) : Switch  Criteria=u2 ~= 0
  rd_addr_counter : hdlsllib/Sources/HDL Counter  CountType=Free running  CountInit=0  CountStep=1  CountMax=255  CountFromType=Initial value  CountFrom=0  CountResetPort=off  CountLoadPort=off  CountEnbPort=on  CountDirPort=off  CountDataType=Unsigned  CountWordLen=ceil(log2(numBins))  CountFracLen=0  CountSampTime=1
      settings: SourceProductName=Simulink
  ramBus : Outport  VectorParamsAs1DForOutWhenUnconnected=off
  excess : Outport  Port=2  VectorParamsAs1DForOutWhenUnconnected=off
  done : Outport  Port=3  VectorParamsAs1DForOutWhenUnconnected=off
  wires:
  Constant/1 -> Switch/1
  totalExcess/1 -> Switch3/3, Shift Arithmetic/1
  Shift Arithmetic/1 -> Add3/1, Add2/2, Add/2
  Constant1/1 -> Switch1/1, Add1/2, Add/1
  Relational Operator/1 -> Switch2/2, Switch1/2
  histoIn/1 -> Add1/3, Add2/1, Relational Operator/1, Compare To Constant/1
  Add/1 -> Relational Operator/2
  Add2/1 -> Switch1/3
  Add1/1 -> Switch2/1
  Add3/1 -> Switch2/3
  Switch1/1 -> Switch/3
  Switch3/1 -> Switch4/1, Add1/1, Add3/2
  Delay/1 -> Switch3/1
  Switch4/1 -> Delay1/1, Delay/1
  Switch2/1 -> Switch4/3
  Delay1/1 -> excess/1
  Delay2/1 -> Delay1/2
  Compare To Constant/1 -> Logical Operator/1
  Logical Operator/1 -> Switch4/2, Switch/2
  Logical Operator1/1 -> Logical Operator/2
  Delay4/1 -> Bus Creator/3  "wr_en"
  Bus Creator/1 -> ramBus/1
  Delay3/1 -> Compare To Constant3/1, Bus Creator/2  "wr_addr"
  Logical Operator3/1 -> Delay2/1, Logical Operator1/1, Switch3/2  "rd_valid"
  Switch/1 -> Bus Creator/1  "histVal"
  rd_addr_counter/1 -> Delay3/1, Bus Creator/4, Compare To Constant2/1  "rd_addr"
  HDL Counter/1 -> Compare To Constant1/1
  Logical Operator2/1 -> Delay4/1, Bus Creator/5, rd_addr_counter/1  "rd_valid"
  Compare To Constant1/1 -> Logical Operator2/2
  Compare To Constant2/1 -> HDL Counter/2
  Compare To Constant3/1 -> Delay5/1, Delay6/1
  Delay5/1 -> done/1
  Delay6/1 -> HDL Counter/1
  active/1 -> Logical Operator3/2, Logical Operator2/1  "rd_valid"
  valid/1 -> Logical Operator3/1  "rd_valid"

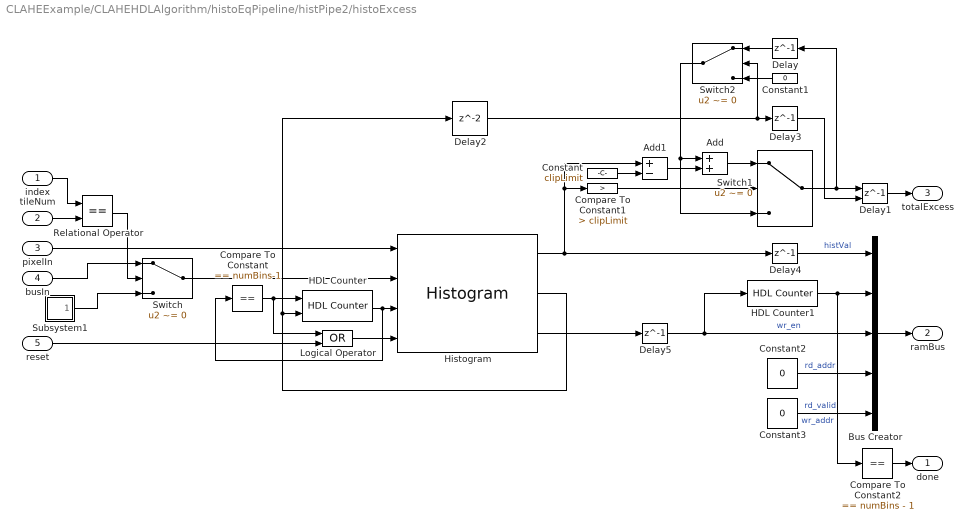
== system CLAHEExample/CLAHEHDLAlgorithm/histoEqPipeline/histPipe2/histoExcess ==
  index : Inport
  tileNum : Inport  Port=2
  pixelIn : Inport  Port=3
  busIn : Inport  Port=4
  reset : Inport  Port=5
  Add : Sum  OutDataTypeStr=fixdt(0,ceil(log2(numPixInTile)),0)
  Add1 : Sum  Inputs=+-
  Bus Creator : BusCreator  Inputs=5
  Compare To Constant : simulink/Logic and Bit Operations/Compare To Constant  relop===  const=numBins-1  OutDataTypeStr=boolean
  Compare To Constant1 : simulink/Logic and Bit Operations/Compare To Constant  relop=>  const=clipLimit  OutDataTypeStr=boolean
  Compare To Constant2 : simulink/Logic and Bit Operations/Compare To Constant  relop===  const=numBins - 1  OutDataTypeStr=boolean
  Constant : Constant  Value=clipLimit  OutDataTypeStr=fixdt(0,ceil(log2(numPixInTile)),0)  SampleTime=-1
  Constant1 : Constant  Value=0  OutDataTypeStr=fixdt(0,ceil(log2(numPixInTile)),0)  SampleTime=-1
  Constant2 : Constant  Value=0  OutDataTypeStr=uint8  SampleTime=-1
  Constant3 : Constant  Value=0  OutDataTypeStr=boolean  SampleTime=-1
  Delay{,3..5} (4 alike) : Delay  DelayLength=1
  Delay1 : Delay  DelayLength=1  ShowEnablePort=on
      settings: InputPortMap=u0,e6
  Delay2 : Delay
  HDL Counter : hdlsllib/Sources/HDL Counter  CountType=Count limited  CountInit=0  CountStep=1  CountMax=numBins-1  CountFromType=Initial value  CountFrom=0  CountResetPort=on  CountLoadPort=off  CountEnbPort=on  CountDirPort=off  CountDataType=Unsigned  CountWordLen=ceil(log2(numBins))  CountFracLen=0  CountSampTime=1
      settings: SourceProductName=Simulink
  HDL Counter1 : hdlsllib/Sources/HDL Counter  CountType=Count limited  CountInit=0  CountStep=1  CountMax=numBins - 1  CountFromType=Initial value  CountFrom=0  CountResetPort=off  CountLoadPort=off  CountEnbPort=on  CountDirPort=off  CountDataType=Unsigned  CountWordLen=ceil(log2(numBins))  CountFracLen=0  CountSampTime=1
      settings: SourceProductName=Simulink
  Histogram : visionhdlstatistics/Histogram  NumBins=256  OutputDataType=Unsigned fixed point  OutputWL=ceil(log2(numPixInTile))  SimulateUsing=Code generation
      settings: SourceProductName=Vision HDL Toolbox  SourceProductBaseCode=VT
  Logical Operator : Logic  Operator=OR  AllPortsSameDT=off  OutDataTypeStr=boolean
  Relational Operator : RelationalOperator  Operator===  OutDataTypeStr=boolean  RndMeth=Nearest
  Subsystem1 : Subsystem
  Switch : Switch  Criteria=u2 ~= 0
  Switch1 : Switch  Criteria=u2 ~= 0
  Switch2 : Switch  Criteria=u2 ~= 0
  done : Outport  VectorParamsAs1DForOutWhenUnconnected=off
  ramBus : Outport  Port=2  VectorParamsAs1DForOutWhenUnconnected=off
  totalExcess : Outport  Port=3  VectorParamsAs1DForOutWhenUnconnected=off
  wires:
  HDL Counter/1 -> Compare To Constant/1, Histogram/3
  Histogram/2 -> Delay2/1, HDL Counter/2
  Delay2/1 -> Switch2/2, Delay3/1
  Logical Operator/1 -> Histogram/4
  Constant/1 -> Add1/2
  Switch1/1 -> Delay1/1, Delay/1
  reset/1 -> Logical Operator/2
  Add/1 -> Switch1/1
  Compare To Constant1/1 -> Switch1/2
  Add1/1 -> Add/2
  Switch2/1 -> Switch1/3, Add/1
  Delay/1 -> Switch2/1
  Histogram/1 -> Delay4/1, Add1/1, Compare To Constant1/1
  Compare To Constant/1 -> Logical Operator/1, HDL Counter/1
  Constant1/1 -> Switch2/3
  pixelIn/1 -> Histogram/1
  Histogram/3 -> Delay5/1
  Delay5/1 -> Bus Creator/3, HDL Counter1/1  "wr_en"
  Delay4/1 -> Bus Creator/1  "histVal"
  HDL Counter1/1 -> Bus Creator/2, Compare To Constant2/1  "wr_addr"
  Constant2/1 -> Bus Creator/4  "rd_addr"
  Constant3/1 -> Bus Creator/5  "rd_valid"
  Bus Creator/1 -> ramBus/1
  Delay1/1 -> totalExcess/1
  Compare To Constant2/1 -> done/1
  busIn/1 -> Switch/1
  Subsystem1/1(Out1) -> Switch/3
  tileNum/1 -> Relational Operator/2
  index/1 -> Relational Operator/1
  Switch/1 -> Histogram/2
  Relational Operator/1 -> Switch/2
  Delay3/1 -> Delay1/2
